simulink model "m030_RoomHeatingSystem"  (R2022a)
settings: Solver=VariableStepAuto  StartTime=0.0  StopTime=24  RelTol=1e-3
settings Model: Creator=Admin  LastModifiedBy=Admin

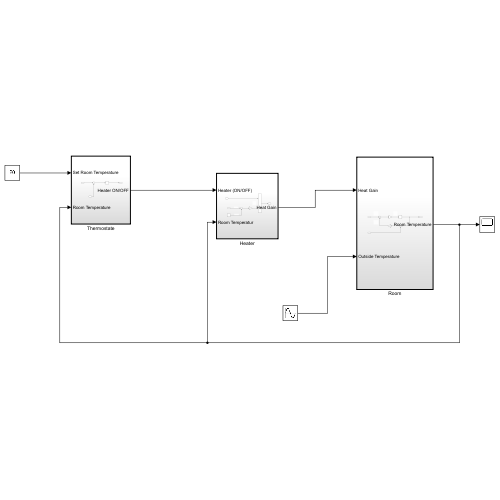
[thumbnail: Simulink's stored preview of the top-level diagram]
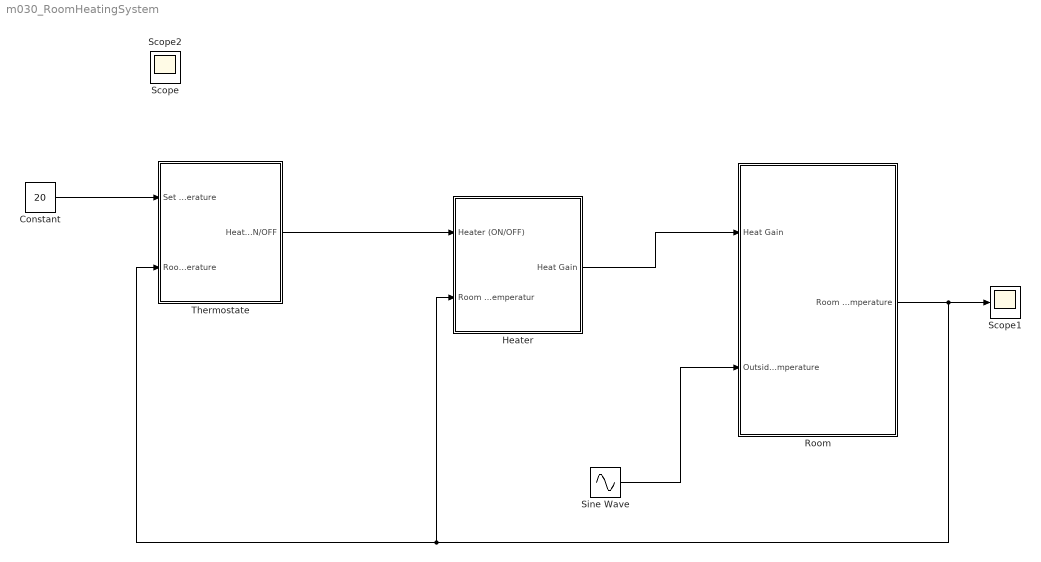
== system m030_RoomHeatingSystem ==
  Constant : Constant  Value=20
  Heater : Subsystem  TreatAsAtomicUnit=on
  Room : Subsystem  TreatAsAtomicUnit=on
  Scope1 : Scope
  Sine Wave : Sin  Amplitude=5  Bias=12  Frequency=2*pi/24  Phase=pi  SampleTime=0
  Thermostate : Subsystem  TreatAsAtomicUnit=on
  Scope : Scope
  Scope2 : Scope
  wires:
  Sine Wave/1 -> Room/2(Outside Temperature)
  Heater/1(Heat Gain) -> Room/1(Heat Gain)
  Room/1(Room Temperature) -> Heater/2(Room Temperatur), Thermostate/2(Room Temperature), Scope1/1
  Constant/1 -> Thermostate/1(Set Room Temperature)
  Thermostate/1(Heater ON/OFF) -> Heater/1(Heater (ON/OFF))

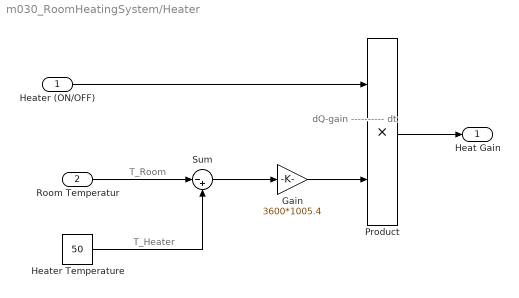
== system m030_RoomHeatingSystem/Heater ==
  note: dQ-gain
      | ----------
      |      dt
  note: T_Room
  note: T_Heater
  Heater (ON/OFF) : Inport
  Room Temperatur : Inport  Port=2
  Gain : Gain  Gain=3600*1005.4
  Heater Temperature : Constant  Value=50
  Product : Product
  Sum : Sum  Inputs=|-+
  Heat Gain : Outport
  wires:
  Room Temperatur/1 -> Sum/1
  Heater Temperature/1 -> Sum/2
  Sum/1 -> Gain/1
  Heater (ON/OFF)/1 -> Product/1
  Gain/1 -> Product/2
  Product/1 -> Heat Gain/1

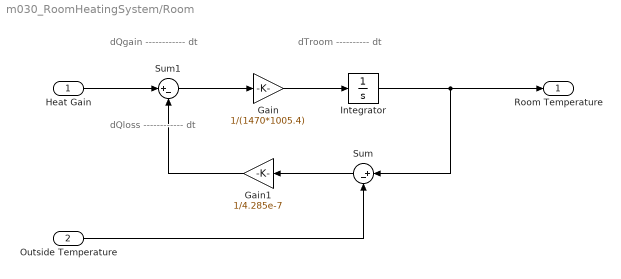
== system m030_RoomHeatingSystem/Room ==
  note: dQgain
      | ------------
      |      dt
  note: dQloss
      | ------------
      |      dt
  note: dTroom
      | ----------
      |     dt
  Heat Gain : Inport
  Outside Temperature : Inport  Port=2
  Gain : Gain  Gain=1/(1470*1005.4)
  Gain1 : Gain  Gain=1/4.285e-7
  Integrator : Integrator  InitialCondition=20
  Sum : Sum  Inputs=|+-
  Sum1 : Sum  Inputs=|+-
  Room Temperature : Outport
  wires:
  Integrator/1 -> Sum/1, Room Temperature/1
  Outside Temperature/1 -> Sum/2
  Sum/1 -> Gain1/1
  Gain1/1 -> Sum1/2
  Heat Gain/1 -> Sum1/1
  Sum1/1 -> Gain/1
  Gain/1 -> Integrator/1

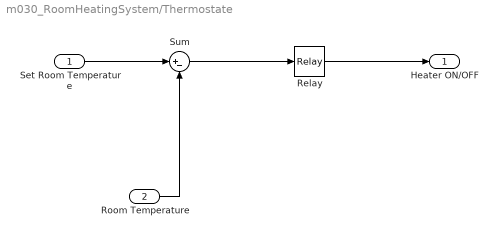
== system m030_RoomHeatingSystem/Thermostate ==
  Set Room Temperature : Inport
  Room Temperature : Inport  Port=2
  Relay : Relay  OnSwitchValue=2  OffSwitchValue=-2
  Sum : Sum  Inputs=|+-
  Heater ON/OFF : Outport
  wires:
  Sum/1 -> Relay/1
  Relay/1 -> Heater ON/OFF/1
  Set Room Temperature/1 -> Sum/1
  Room Temperature/1 -> Sum/2
